simulink model "bezObserwatora"  (R2022b)
settings: Solver=ode4  StartTime=0.0  StopTime=tSim  FixedStep=h  RelTol=1e-3
values from neighbouring files (symbols this model uses):
  K = lqr(system, Q, R)    [main.m]
  params = [M, m, L, b, g, I]    [main.m]
  state0 = [x0, xDot0, theta0, thetaDot0]    [main.m]
  Y = [y, 0, 0, 0]'    [main.m]
settings Model: Creator=asialalala  LastModifiedBy=asialalala
settings DataIOCC: SaveFormat=Array  ReturnWorkspaceOutputs=off

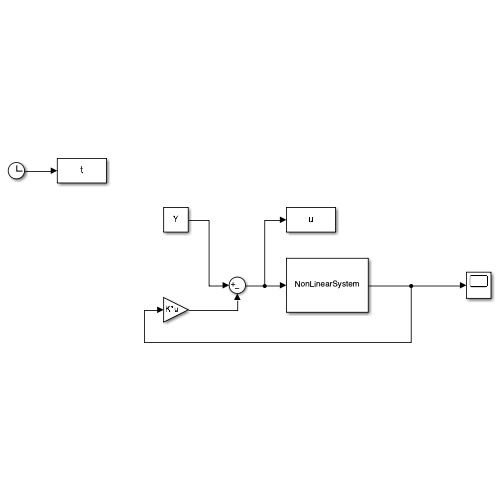
[thumbnail: Simulink's stored preview of the top-level diagram]
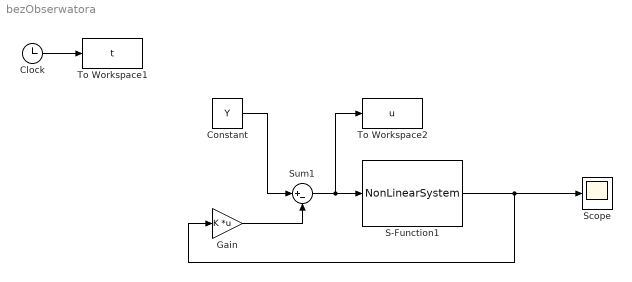
== system bezObserwatora ==
  Clock : Clock
  Constant : Constant  Value=Y
  Gain : Gain  Gain=K  Multiplication=Matrix(K*u)
  S-Function1 : S-Function  FunctionName=NonLinearSystem  Parameters=state0,params  SFunctionDeploymentMode=off  EnableBusSupport=off
  Scope : Scope
  Sum1 : Sum  Inputs=|+-
  To Workspace1 : ToWorkspace  VariableName=t  SampleTime=-1
  To Workspace2 : ToWorkspace  VariableName=u  SampleTime=-1
  wires:
  S-Function1/1 -> Gain/1, Scope/1
  Clock/1 -> To Workspace1/1
  Constant/1 -> Sum1/1
  Gain/1 -> Sum1/2
  Sum1/1 -> To Workspace2/1, S-Function1/1
